simulink model "JonasTrafficLightController"  (R2020a)
settings: Solver=FixedStepAuto  StartTime=0.0  StopTime=120  FixedStep=1  RelTol=1e-3
settings Model: EnablePacing=on  Creator=Aashkaran Dhillon  LastModifiedBy=Aashkaran Dhillon

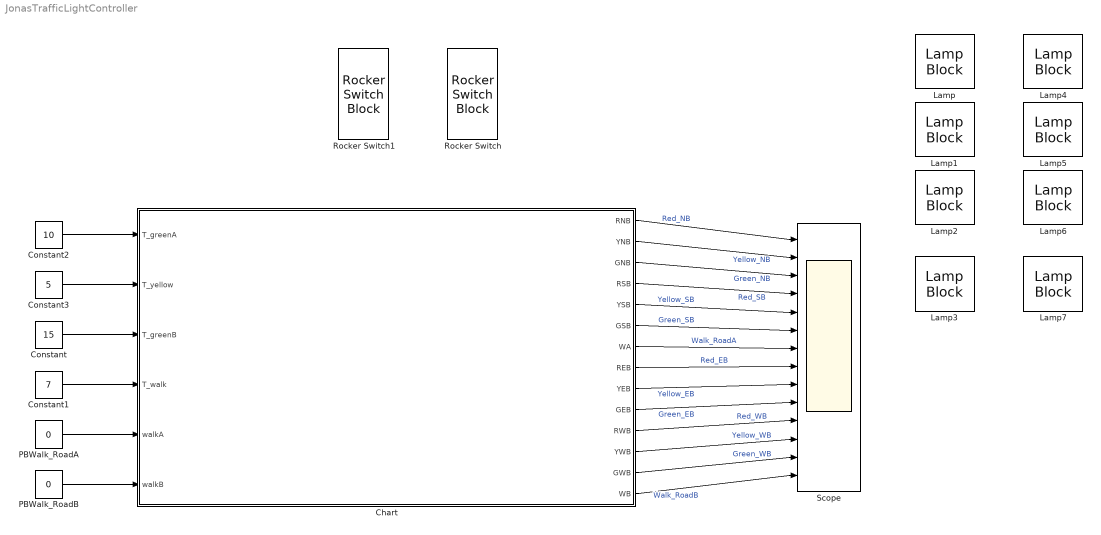
== system JonasTrafficLightController ==
  Chart : Stateflow chart  TreatAsAtomicUnit=on
      settings: PortSchema="{\"entries\":[{\"content\":{\"sides\":[{\"content\":{\"connectorIds\":[\"In1\",\"In3\",\"In2\",\"In4\",\"In5\",\"In6\"]},\"type\":\"ConnectorPlacement.EquallySpacedRectSide\",\"uuid\":\"1cefa32e-2f89-4dce-8e58-63bf26535dfd\"},{\"content\":{\"connectorIds\":[\"Out1\",\"Out2\",\"Out3\",\"Out4\",\"Out5\",\"Out6\",\"Out7\",\"Out8\",\"Out9\",\"Out10\",\"Out11\",\"Out12\",\"Out13\",\"Out14\"],\"side\":\"RIGHT\"},\"type\":\"ConnectorPlacement.EquallySpacedRectSide\",\"uuid\":\"ee62f933-101b-40b6-a0a7-a59b15cd1a2f\"},{\"content\":{\"connectorIds\":[],\"side\":\"TOP\"},\"type\":\"ConnectorPlacement.EquallySpacedRectSide\",\"uuid\":\"be8bbc96-3190-455a-ba46-a9efc56ab94f\"}]},\"type\":\"ConnectorPlacement.EquallySpacedConnector\",\"uuid\":\"ab6252b4-e5c5-42a1-8b00-e9ea8abf8852\"}],\"packageUris\":[\"http://schema.mathworks.com/mf0/Connector/19700101\"],\"version\":\"1.0\"}"
  Constant : Constant  Value=15
  Constant1 : Constant  Value=7
  Constant2 : Constant  Value=10
  Constant3 : Constant  Value=5
  Lamp{,1..7} (8 alike) : LampBlock
      Lamp3 settings: AttributesFormatString=Walk Road A
      Lamp7 settings: AttributesFormatString=Walk Road B
  PBWalk_RoadA : Constant  Value=0
  PBWalk_RoadB : Constant  Value=0
  Rocker Switch : RockerSwitchBlock
      settings: Values={{'Off', 'On'}, [0 1]}
  Rocker Switch1 : RockerSwitchBlock
      settings: Values={{'Off', 'On'}, [0 1]}
  Scope : Scope  NumInputPorts=14
  wires:
  Constant/1 -> Chart/2(T_greenB)
  Chart/3(GNB) -> Scope/3  "Green_NB"
  Chart/4(RSB) -> Scope/4  "Red_SB"
  Chart/5(YSB) -> Scope/5  "Yellow_SB"
  Chart/6(GSB) -> Scope/6  "Green_SB"
  Chart/7(WA) -> Scope/7  "Walk_RoadA"
  Chart/8(REB) -> Scope/8  "Red_EB"
  Chart/9(YEB) -> Scope/9  "Yellow_EB"
  Chart/10(GEB) -> Scope/10  "Green_EB"
  Chart/11(RWB) -> Scope/11  "Red_WB"
  Chart/12(YWB) -> Scope/12  "Yellow_WB"
  Chart/13(GWB) -> Scope/13  "Green_WB"
  Chart/14(WB) -> Scope/14  "Walk_RoadB"
  Chart/2(YNB) -> Scope/2  "Yellow_NB"
  Chart/1(RNB) -> Scope/1  "Red_NB"
  Constant2/1 -> Chart/1(T_greenA)
  PBWalk_RoadB/1 -> Chart/6(walkB)
  PBWalk_RoadA/1 -> Chart/5(walkA)
  Constant1/1 -> Chart/4(T_walk)
  Constant3/1 -> Chart/3(T_yellow)

== stateflow chart JonasTrafficLightController/Chart ==
  state walkA
    entry:
    [WA,WB]=deal(1,0);
    on after(T_walk,sec):
    [WA,WB]=deal(0,0);
  state S02
    entry:
    [RNB,YNB,GNB]=deal(1,0,0);
    [RSB,YSB,GSB]=deal(1,0,0);
    [REB,YEB,GEB]=deal(0,0,1);
    [RWB,YWB,GWB]=deal(0,0,1);
    [WA,WB]=deal(0,0);
  state S01
    entry:
    [RNB,YNB,GNB]=deal(0,1,0);
    [RSB,YSB,GSB]=deal(0,1,0);
    [REB,YEB,GEB]=deal(1,0,0);
    [RWB,YWB,GWB]=deal(1,0,0);
    [WA,WB]=deal(0,0);
  state S00
    entry:
    [RNB,YNB,GNB]=deal(0,0,1);
    [RSB,YSB,GSB]=deal(0,0,1);
    [REB,YEB,GEB]=deal(1,0,0);
    [RWB,YWB,GWB]=deal(1,0,0);
    [WA,WB]=deal(0,0);
  state S03
    entry:
    [RNB,YNB,GNB]=deal(1,0,0);
    [RSB,YSB,GSB]=deal(1,0,0);
    [REB,YEB,GEB]=deal(0,1,0);
    [RWB,YWB,GWB]=deal(0,1,0);
    [WA,WB]=deal(0,0);
  state walkB
    entry:
    [WA,WB]=deal(0,1);
    on after(T_walk,sec):
    [WA,WB]=deal(0,0);
  (junction 77) -> walkA [order 2] : [walkA==1]
  walkA -> S01 : [after(T_greenB,sec)]
  (default) -> S00
  S01 -> S02 : [after(T_yellow,sec)]
  S00 -> (junction 77)
  (junction 77) -> S01 [order 1] : after(T_greenB,sec)
  S03 -> S00 : [after(T_yellow,sec)]
  S02 -> (junction 75)
  (junction 75) -> S03 [order 2] : [after(T_greenA,sec)]
  (junction 75) -> walkB [order 1] : [walkB==1]
  walkB -> S03 : [after(T_greenA,sec)]
  data: T_greenA input; T_greenB input; T_yellow input =5; T_walk input =30; walkA input; RNB output; YNB output; GNB output; RSB output; YSB output; GSB output; WA output; REB output; YEB output; GEB output; RWB output; YWB output; GWB output; WB output; walkB input
